simulink model "Practica2_ejercicio1"  (R2012b)
settings: Solver=ode45  StartTime=0.0  StopTime=20  RelTol=1e-3
values from neighbouring files (symbols this model uses):
  C = Ch*inv(D)    [invhomo.m]
undefined symbols (not defined in the file or in its folder): L, R
settings Model: Creator=isa  LastModifiedBy=isa

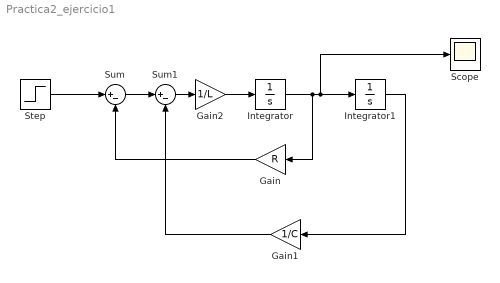
== system Practica2_ejercicio1 ==
  Gain : Gain  Gain=R
  Gain1 : Gain  Gain=1/C
  Gain2 : Gain  Gain=1/L
  Integrator : Integrator
  Integrator1 : Integrator
  Scope : Scope
  Step : Step  SampleTime=0
  Sum : Sum  Inputs=|+-
  Sum1 : Sum  Inputs=|+-
  wires:
  Integrator1/1 -> Gain1/1
  Step/1 -> Sum/1
  Gain/1 -> Sum/2
  Sum/1 -> Sum1/1
  Gain1/1 -> Sum1/2
  Integrator/1 -> Gain/1, Scope/1, Integrator1/1
  Sum1/1 -> Gain2/1
  Gain2/1 -> Integrator/1
